simulink model "HDLTxRx"  (R2024a)
settings: Solver=FixedStepDiscrete  StartTime=0.0  StopTime=stopTime  RelTol=1e-3
values from neighbouring files (symbols this model uses):
  delayIn = 1000    [testTxRx.m]
  pWords = binl2str(pBits)    [testTxRx.m]
undefined symbols (not defined in the file or in its folder): fPHY, payloadLenInFecBlocks
libraries: dspsrcs4 x6, hdlsllib x3, HDL_ieee_8021513 x3, whdlutilities x1
settings Model: DataTypeOverride=Off  SimulationMode=accelerator  Creator=cotti  LastModifiedBy=cotti
settings OptimizationCC: BlockReduction=off  ConditionallyExecuteInputs=off  DefaultParameterBehavior=Inlined  InheritOutputTypeSmallerThanSingle=on
settings DebuggingCC: ArtificialAlgebraicLoopMsg=error  SingleTaskRateTransMsg=error
settings HardwareCC: ProdBitPerPointer=32  ProdBitPerSizeT=32  ProdBitPerPtrDiffT=32  ProdLargestAtomicFloat=None  ProdIntDivRoundTo=Undefined  ProdEndianess=Unspecified  ProdWordSize=32  ProdHWDeviceType=ASIC/FPGA->ASIC/FPGA  TargetBitPerLong=64  TargetBitPerPointer=64  TargetBitPerSizeT=64  TargetBitPerPtrDiffT=64  TargetLongLongMode=on  TargetIntDivRoundTo=Zero  TargetEndianess=LittleEndian  TargetWordSize=64  TargetHWDeviceType=Custom Processor->MATLAB Host Computer  ProdEqTarget=off

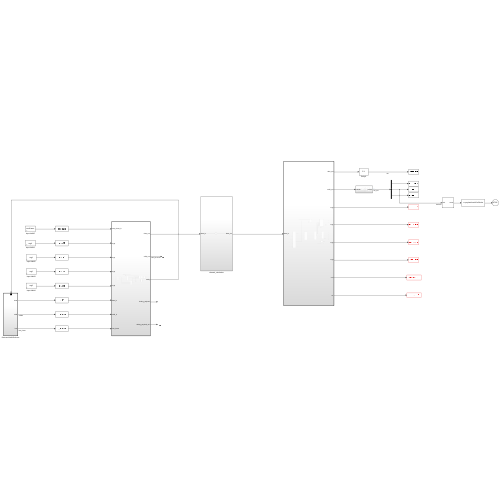
[thumbnail: Simulink's stored preview of the top-level diagram]
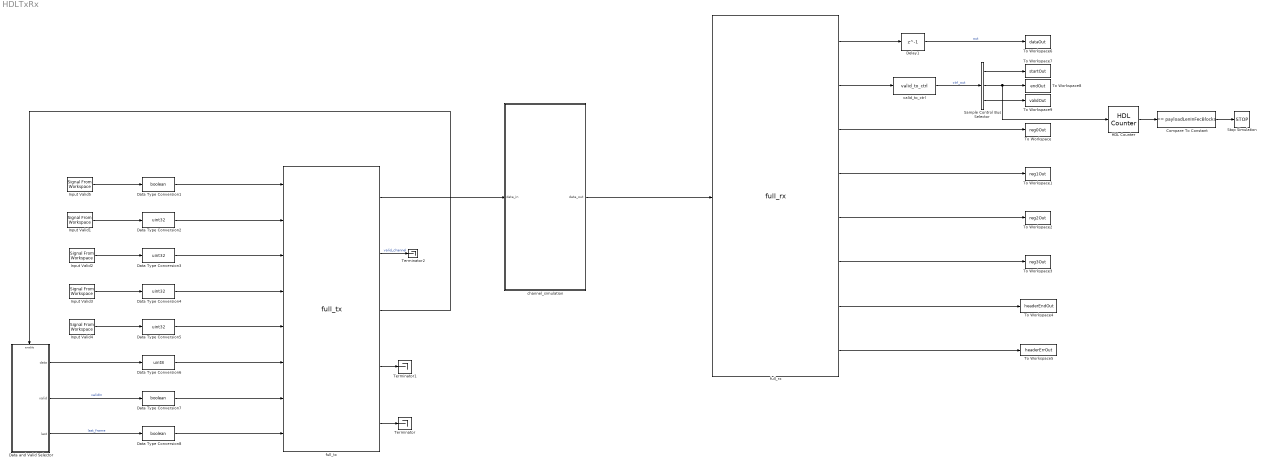
== system HDLTxRx ==
  Compare To Constant : hdlsllib/Logic and Bit Operations/Compare To Constant  relop===  const=payloadLenInFecBlocks  OutDataTypeStr=boolean
  Data Type Conversion1 : DataTypeConversion  OutDataTypeStr=boolean  SaturateOnIntegerOverflow=off  RndMeth=Floor
  Data Type Conversion{2..5} (4 alike) : DataTypeConversion  OutDataTypeStr=uint32  SaturateOnIntegerOverflow=off  RndMeth=Floor
  Data Type Conversion6 : DataTypeConversion  OutDataTypeStr=uint8  SaturateOnIntegerOverflow=off  RndMeth=Floor
  Data Type Conversion7 : DataTypeConversion  OutDataTypeStr=boolean  SaturateOnIntegerOverflow=off  RndMeth=Floor
  Data Type Conversion8 : DataTypeConversion  OutDataTypeStr=boolean  SaturateOnIntegerOverflow=off  RndMeth=Floor
  Data and Valid Selector : Subsystem  TreatAsAtomicUnit=on
  Delay1 : Delay  DelayLength=1  InitialCondition=0  UseCircularBuffer=on
  HDL Counter : hdlsllib/Sources/HDL Counter  CountType=Free running  CountInit=0  CountStep=1  CountMax=25  CountFromType=Initial value  CountFrom=0  CountResetPort=off  CountLoadPort=off  CountEnbPort=on  CountDirPort=off  CountHitOutputPort=off  CountDataType=Unsigned  CountWordLen=32  CountFracLen=0  CountSampTime=1
  Input Valid1 : dspsrcs4/Signal From Workspace  X=reg0  Ts=1/(fPHY/4)  nsamps=1  OutputAfterFinalValue=Setting to zero  ignoreOrWarnInputAndFrameLengths=off  OutputFrames=off
  Input Valid2 : dspsrcs4/Signal From Workspace  X=reg1  Ts=1/(fPHY/4)  nsamps=1  OutputAfterFinalValue=Setting to zero  ignoreOrWarnInputAndFrameLengths=off  OutputFrames=off
  Input Valid3 : dspsrcs4/Signal From Workspace  X=reg2  Ts=1/(fPHY/4)  nsamps=1  OutputAfterFinalValue=Setting to zero  ignoreOrWarnInputAndFrameLengths=off  OutputFrames=off
  Input Valid4 : dspsrcs4/Signal From Workspace  X=reg3  Ts=1/(fPHY/4)  nsamps=1  OutputAfterFinalValue=Setting to zero  ignoreOrWarnInputAndFrameLengths=off  OutputFrames=off
  Input Valid5 : dspsrcs4/Signal From Workspace  X=newFrame  Ts=1/(fPHY/4)  nsamps=1  OutputAfterFinalValue=Setting to zero  ignoreOrWarnInputAndFrameLengths=off  OutputFrames=off
  Sample Control Bus Selector : whdlutilities/Sample Control Bus Selector  OutputSignals=start,end,valid
  Stop Simulation : Stop
  Terminator : Terminator
  Terminator1 : Terminator
  Terminator2 : Terminator
  To Workspace : ToWorkspace  VariableName=reg0Out  SampleTime=4/fPHY
      settings: Save2DSignal=2-D array (concatenate along first dimension)
  To Workspace1 : ToWorkspace  VariableName=reg1Out  SampleTime=4/fPHY
      settings: Save2DSignal=2-D array (concatenate along first dimension)
  To Workspace2 : ToWorkspace  VariableName=reg2Out  SampleTime=4/fPHY
      settings: Save2DSignal=2-D array (concatenate along first dimension)
  To Workspace3 : ToWorkspace  VariableName=reg3Out  SampleTime=4/fPHY
      settings: Save2DSignal=2-D array (concatenate along first dimension)
  To Workspace4 : ToWorkspace  VariableName=headerEndOut  SampleTime=4/fPHY
      settings: Save2DSignal=2-D array (concatenate along first dimension)
  To Workspace5 : ToWorkspace  VariableName=headerErrOut  SampleTime=4/fPHY
      settings: Save2DSignal=2-D array (concatenate along first dimension)
  To Workspace6 : ToWorkspace  VariableName=dataOut  SampleTime=2/fPHY
      settings: Save2DSignal=2-D array (concatenate along first dimension)
  To Workspace7 : ToWorkspace  VariableName=startOut  SampleTime=2/fPHY
      settings: Save2DSignal=2-D array (concatenate along first dimension)
  To Workspace8 : ToWorkspace  VariableName=endOut  SampleTime=2/fPHY
      settings: Save2DSignal=2-D array (concatenate along first dimension)
  To Workspace9 : ToWorkspace  VariableName=validOut  SampleTime=2/fPHY
      settings: Save2DSignal=2-D array (concatenate along first dimension)
  channel_simulation : Subsystem
  full_rx : HDL_ieee_8021513/full_rx  SystemSampleTime=-1  VariantActivationTime=update diagram  AllowFlexibleInterface=on  Latency=0  AutoFrameSizeCalculation=off
      settings: SourceProductName=HDL IEEE 8021513
  full_tx : HDL_ieee_8021513/full_tx  SystemSampleTime=-1  VariantActivationTime=update diagram  AllowFlexibleInterface=on  Latency=0  AutoFrameSizeCalculation=off
      settings: SourceProductName=HDL IEEE 8021513
  valid_to_ctrl : HDL_ieee_8021513/valid_to_ctrl  SystemSampleTime=-1  VariantActivationTime=update diagram  AllowFlexibleInterface=on  Latency=0  AutoFrameSizeCalculation=off
      settings: SourceProductName=HDL IEEE 8021513
  wires:
  full_tx/5 -> Terminator/1
  full_tx/4 -> Terminator1/1
  Input Valid1/1 -> Data Type Conversion2/1
  Input Valid4/1 -> Data Type Conversion5/1
  Data Type Conversion8/1 -> full_tx/8
  Data and Valid Selector/3(last) -> Data Type Conversion8/1  "last_frame"
  Data Type Conversion4/1 -> full_tx/4
  Data Type Conversion3/1 -> full_tx/3
  Data Type Conversion2/1 -> full_tx/2
  Input Valid5/1 -> Data Type Conversion1/1
  Input Valid3/1 -> Data Type Conversion4/1
  Data and Valid Selector/1(data) -> Data Type Conversion6/1
  Data Type Conversion1/1 -> full_tx/1
  Input Valid2/1 -> Data Type Conversion3/1
  Data Type Conversion5/1 -> full_tx/5
  Data Type Conversion6/1 -> full_tx/6
  Data Type Conversion7/1 -> full_tx/7
  Data and Valid Selector/2(valid) -> Data Type Conversion7/1  "validIn"
  full_tx/3 -> Data and Valid Selector/Enable
  full_tx/1 -> channel_simulation/1(data_in)
  full_rx/6 -> To Workspace3/1
  full_rx/8 -> To Workspace5/1
  Sample Control Bus Selector/1 -> To Workspace7/1
  Delay1/1 -> To Workspace6/1  "out"
  full_rx/7 -> To Workspace4/1
  full_rx/1 -> Delay1/1
  valid_to_ctrl/1 -> Sample Control Bus Selector/1  "ctrl_out"
  Sample Control Bus Selector/3 -> To Workspace9/1
  full_rx/5 -> To Workspace2/1
  full_rx/3 -> To Workspace/1
  full_rx/2 -> valid_to_ctrl/1
  full_rx/4 -> To Workspace1/1
  full_tx/2 -> Terminator2/1  "valid_channel"
  channel_simulation/1(data_out) -> full_rx/1
  HDL Counter/1 -> Compare To Constant/1
  Sample Control Bus Selector/2 -> HDL Counter/1, To Workspace8/1
  Compare To Constant/1 -> Stop Simulation/1

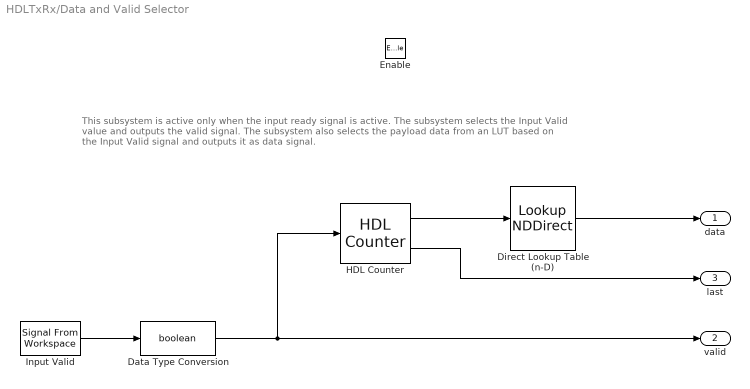
== system HDLTxRx/Data and Valid Selector ==
  note: This subsystem is active only when the input ready signal is active. The subsystem selects the Input Valid value and outputs the valid signal.
      | The subsystem also selects the payload data from an LUT based on the Input Valid signal and outputs it as data signal.
  Enable : EnablePort
  Data Type Conversion : DataTypeConversion  OutDataTypeStr=boolean  SaturateOnIntegerOverflow=off  RndMeth=Floor
  Direct Lookup Table (n-D) : LookupNDDirect  NumberOfTableDimensions=1  Table=uint8(pWords')  DiagnosticForOutOfRangeInput=Error  TableDataTypeStr=uint8
  HDL Counter : hdlsllib/Sources/HDL Counter  CountType=Count limited  CountInit=0  CountStep=1  CountMax=length(pWords) -1  CountFromType=Initial value  CountFrom=0  CountResetPort=off  CountLoadPort=off  CountEnbPort=on  CountDirPort=off  CountHitOutputPort=on  CountDataType=Unsigned  CountWordLen=nextpow2(length(pWords))  CountFracLen=0  CountSampTime=1
  Input Valid : dspsrcs4/Signal From Workspace  X=validIn  Ts=1/(fPHY/4)  nsamps=1  OutputAfterFinalValue=Setting to zero  ignoreOrWarnInputAndFrameLengths=off  OutputFrames=off
  data : Outport  InitialOutput=0  VectorParamsAs1DForOutWhenUnconnected=off
  valid : Outport  Port=2  InitialOutput=0  VectorParamsAs1DForOutWhenUnconnected=off
  last : Outport  Port=3  VectorParamsAs1DForOutWhenUnconnected=off
  wires:
  HDL Counter/1 -> Direct Lookup Table (n-D)/1
  Direct Lookup Table (n-D)/1 -> data/1
  HDL Counter/2 -> last/1
  Input Valid/1 -> Data Type Conversion/1
  Data Type Conversion/1 -> valid/1, HDL Counter/1

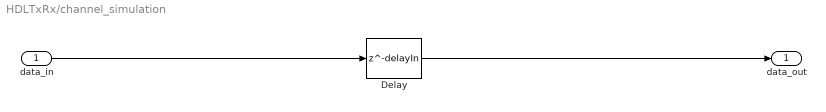
== system HDLTxRx/channel_simulation ==
  data_in : Inport
  Delay : Delay  DelayLength=delayIn  InitialCondition=0  UseCircularBuffer=on
  data_out : Outport
  wires:
  data_in/1 -> Delay/1
  Delay/1 -> data_out/1
